simulink library "UserBlocks"  (R2014a)
settings: Solver=ode45  SolverMode=SingleTasking  StartTime=0.0  StopTime=10.0  RelTol=1e-3
values from neighbouring files (symbols this model uses):
  a = param.a    [DSC_Control_Analysis.m]    (also in DSC_Control_Analysis_Exp.m; DSC_Speed_Control_Analysis.m; EmpiricalTireCurves.m = 1.35; FFW_Fx.m = sqrt(curvature/(2*clothoidLength)))
  b = 1.15    [EmpiricalTireCurves.m]
  Cfls = Cfl    [EC_params_nissan.m]
  Crls = Crl    [EC_params_nissan.m]
  d0 = CSTR.d0    [Ext_MPCPara.m]
  freq = Fs/2*linspace(0,1,NFFT/2)    [AACplottingcode.m]    (also in If_alpha_tp_observer.m; If_alpha_tp_observer_for_c_code.m; If_alpha_tp_observer_shoreline.m)
  Iz = param.Iz    [DSC_Control_Analysis.m]    (also in DSC_Control_Analysis_Exp.m; DSC_Speed_Control_Analysis.m; EmpiricalTireCurves.m = 1300)
  K = 10    [EC_params_nissan.m]
  Ks = -10    [EC_params_nissan.m]
  Ksl = -10    [EC_params_nissan.m]
  Kt = 40000    [EC_params_nissan.m]
  Ku = -40000    [EC_params_nissan.m]
  m = 1724    [EmpiricalTireCurves.m]
  mu_s = mu_p    (= 0.6)    [EC_params_nissan.m]    (also in EmpiricalTireCurves.m = 0.55)
  Ns = 10    [EC_params_nissan.m]
  num = num+MTnum(m)    [Build_MtMuMy.m]
  q = 1    [EC_params_nissan.m]
  Taoh = CSTR.Taoh    [Ext_MPCPara.m]
  Ts = 0.002    [DSC_Control_Analysis.m]    (also in DSC_Control_Analysis_Exp.m; DSC_Speed_Control_Analysis.m; EC_params_nissan.m; Ext_MPCPara.m = SSD.Ts)
undefined symbols (not defined in the file or in its folder): acceAmp, ack, alphaFrontSteeringLimit, alphaFrontTable, bit, c, Cfl, Crl, CSTR, dden, deltaPsiDotGain, deltDist, den, denafilt, dnum, elaDotGain, filtera, filterb, frontAlphaLookup, frontForceLookup, FuelStartCalTime, FyFtable, gpsins, h, h_roll, hal_filter_den, hal_filter_num, hwx, hwy5, initAcce, initSpeed, isDriverNoise, lkparams, mapDataFull, mapMatchingParams, maxFrontForce, maxNumSegs, mdPtrs, numafilt, param, rearAlphaLookup, rfl, rfr, rrl, rrr, sglu, SIMP, simuCond, slimFxl, slimFxu, sliml, slimMll, slimMlr, slimMul, slimMur, slimu, sr, SSD, Standard, steering_limit ... (+7)
libraries: simulink x28, slrtlib x18, UserBlocks x6, slrtsoftinglib x6, MickLibBlocks x1, DriftControllerLibrary x1
(part 5 of 6)

== system UserBlocks/MPCACC/PIDACC/MPC MTCACC/MTC ACC control ==
  mdPtrs : Inport
  sysOuts : Inport  Port=2
  Prevel : Inport  Port=3
  VehVel : Inport  Port=4
  MPC CAN Receive1 : Subsystem  AncestorBlock=UserBlocks/MPC CAN Connection/MPC CAN Receive
  MPC CAN Send : Subsystem  AncestorBlock=UserBlocks/MPC CAN Connection/MPC CAN Send
  Samp2 : ZeroOrderHold  SampleTime=SSD.Ts
  Samp4 : ZeroOrderHold  SampleTime=SSD.Ts
  "Setup " : slrtsoftinglib/CAN-AC2-104 SJA 1000/Setup   board=1  can1Baudrate=500 kBaud  can1UserBR=[1,1,4,3]  can2Baudrate=500 kBaud  can2UserBR=[1,1,4,3]  init=[]  term=[]  bus_off_out=off  bus_off_rec=Off  ioBaseAddressL=0x240  memBaseAddressL=0xd0000  intNo=None
  T : Terminator
  Unit Delay : UnitDelay  SampleTime=SSD.Ts
  Ctrl : Outport
  epsilon : Outport  Port=2
  wires:
  MPC CAN Receive1/1(Ctrl) -> Ctrl/1, Unit Delay/1  "u(k)"
  MPC CAN Receive1/2(epsilon) -> epsilon/1
  Prevel/1 -> Samp4/1
  sysOuts/1 -> MPC CAN Send/2(sysOuts)
  VehVel/1 -> Samp2/1
  Unit Delay/1 -> MPC CAN Send/3(Ctrl)
  Samp4/1 -> MPC CAN Send/4(Prevel)
  Samp2/1 -> T/1
  mdPtrs/1 -> MPC CAN Send/1(mdPtrs)

== system UserBlocks/Steering Controller/HAL-9000/Double chirp/Chirp One ==
  note: freqSlope = deltaFreq/targetTime;
      | instantaneousFreq(t) = freqSlope*t + initialFreq;
      | intantaneousPhase(t) = integral(instFreq) = ...
      |       0.5*freqSlope*t^2 + initialFreq*t;
      | outputSignal(t) = sin(instantaneousPhase(t));
  Start Time : Inport
  Clock1 : Clock
      settings: DisableCoverage=on
  Gain : Gain  DisableCoverage=on  Gain=0.5  OutDataTypeStr=Inherit: Same as input  ParamDataTypeStr=Inherit: Same as input
  Output : Trigonometry
  Product : Product  DisableCoverage=on  Inputs=*/  SaturateOnIntegerOverflow=on  InputSameDT=on  OutDataTypeStr=Inherit: Same as first input
  Product1 : Product  DisableCoverage=on  SaturateOnIntegerOverflow=on  InputSameDT=on  OutDataTypeStr=Inherit: Same as first input
  Product2 : Product  DisableCoverage=on  SaturateOnIntegerOverflow=on  InputSameDT=on  OutDataTypeStr=Inherit: Same as first input
  Saturation : Saturate  UpperLimit=duration/2  LowerLimit=0
  Sum : Sum  DisableCoverage=on  Inputs=|++  SaturateOnIntegerOverflow=on  InputSameDT=on  OutDataTypeStr=Inherit: Same as first input
  Sum1 : Sum  DisableCoverage=on  Inputs=-+|  SaturateOnIntegerOverflow=on  InputSameDT=on  OutDataTypeStr=Inherit: Same as first input
  deltaFreq : Constant  DisableCoverage=on  Value=2*pi*(f2-f1)
  initialFreq : Constant  DisableCoverage=on  Value=2*pi*f1
  targetTime : Constant  DisableCoverage=on  Value=T
  Out2 : Outport
  wires:
  Saturation/1 -> Product2/1, Product1/1
  Output/1 -> Out2/1
  Product2/1 -> Output/1
  Sum/1 -> Product2/2
  initialFreq/1 -> Sum/2
  Product1/1 -> Sum/1
  Gain/1 -> Product1/2
  Product/1 -> Gain/1
  targetTime/1 -> Product/2
  deltaFreq/1 -> Product/1
  Start Time/1 -> Sum1/1
  Clock1/1 -> Sum1/2
  Sum1/1 -> Saturation/1

== system UserBlocks/Steering Controller/HAL-9000/Double chirp/Chirp Two ==
  note: freqSlope = deltaFreq/targetTime;
      | instantaneousFreq(t) = freqSlope*t + initialFreq;
      | intantaneousPhase(t) = integral(instFreq) = ...
      |       0.5*freqSlope*t^2 + initialFreq*t;
      | outputSignal(t) = sin(instantaneousPhase(t));
  Start Time : Inport
  Clock1 : Clock
      settings: DisableCoverage=on
  Gain : Gain  DisableCoverage=on  Gain=0.5  OutDataTypeStr=Inherit: Same as input  ParamDataTypeStr=Inherit: Same as input
  Output : Trigonometry
  Product : Product  DisableCoverage=on  Inputs=*/  SaturateOnIntegerOverflow=on  InputSameDT=on  OutDataTypeStr=Inherit: Same as first input
  Product1 : Product  DisableCoverage=on  SaturateOnIntegerOverflow=on  InputSameDT=on  OutDataTypeStr=Inherit: Same as first input
  Product2 : Product  DisableCoverage=on  SaturateOnIntegerOverflow=on  InputSameDT=on  OutDataTypeStr=Inherit: Same as first input
  Saturation : Saturate  UpperLimit=duration/2  LowerLimit=0
  Sum : Sum  DisableCoverage=on  Inputs=|++  SaturateOnIntegerOverflow=on  InputSameDT=on  OutDataTypeStr=Inherit: Same as first input
  Sum1 : Sum  DisableCoverage=on  Inputs=-+|  SaturateOnIntegerOverflow=on  InputSameDT=on  OutDataTypeStr=Inherit: Same as first input
  deltaFreq : Constant  DisableCoverage=on  Value=2*pi*(f2-f1)
  initialFreq : Constant  DisableCoverage=on  Value=2*pi*f1
  targetTime : Constant  DisableCoverage=on  Value=T
  Out2 : Outport
  wires:
  Saturation/1 -> Product2/1, Product1/1
  Output/1 -> Out2/1
  Product2/1 -> Output/1
  Sum/1 -> Product2/2
  initialFreq/1 -> Sum/2
  Product1/1 -> Sum/1
  Gain/1 -> Product1/2
  Product/1 -> Gain/1
  targetTime/1 -> Product/2
  deltaFreq/1 -> Product/1
  Start Time/1 -> Sum1/1
  Clock1/1 -> Sum1/2
  Sum1/1 -> Saturation/1

== system UserBlocks/TTS Steering Control/Compute Steering Along Path/StaticMap/Map-Matching Primatives Dynamic Map P1 ==
  States : Inport
  Map : Inport  Port=2
  3-second delay : Step  Time=3  SampleTime=0
  Bus Creator : BusCreator  Inputs=3
  Bus Selector : BusSelector  OutputSignals=Pos E,Pos N,Yaw Angle,Vx
  Constant : Constant  Value=0
  Constant1 : Constant  Value=pi/2  SampleTime=Ts
  Data Type Conversion : DataTypeConversion  OutDataTypeStr=double
  General Map-Matching Dynamic Map : Subsystem
  Logical Operator : Logic  Operator=OR  AllPortsSameDT=off  OutDataTypeStr=boolean
  Sum : Sum  Inputs=|++
  Unit Delay : UnitDelay  SampleTime=-1
  Match Out : Outport
  wires:
  Constant/1 -> General Map-Matching Dynamic Map/3(posU)
  Logical Operator/1 -> Data Type Conversion/1, Unit Delay/1
  Bus Selector/3 -> Sum/1  "<Yaw Angle>"
  Data Type Conversion/1 -> General Map-Matching Dynamic Map/6(enable)
  Unit Delay/1 -> Logical Operator/2
  3-second delay/1 -> Logical Operator/1
  Bus Selector/4 -> General Map-Matching Dynamic Map/5(vx_cg)  "<Vx>"
  General Map-Matching Dynamic Map/3(debugOut) -> Bus Creator/3  "debugOut"
  Sum/1 -> General Map-Matching Dynamic Map/4(yaw)
  Constant1/1 -> Sum/2
  General Map-Matching Dynamic Map/2(curOut) -> Bus Creator/2  "curOut"
  General Map-Matching Dynamic Map/1(matchOut) -> Bus Creator/1  "matchOut"
  States/1 -> Bus Selector/1
  Bus Selector/1 -> General Map-Matching Dynamic Map/1(posE)  "<Pos E>"
  Bus Selector/2 -> General Map-Matching Dynamic Map/2(posN)  "<Pos N>"
  Bus Creator/1 -> Match Out/1
  Map/1 -> General Map-Matching Dynamic Map/7(Map)

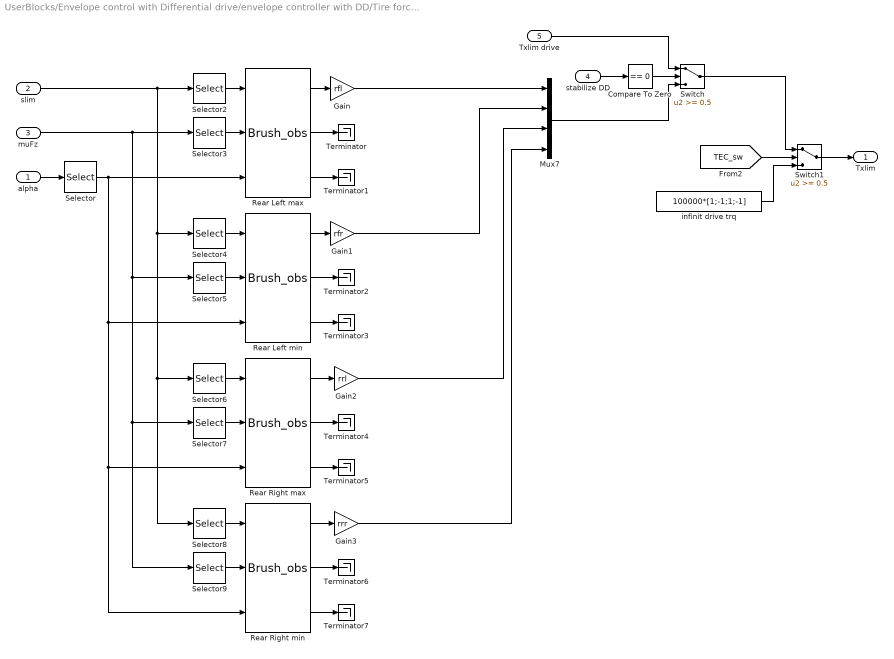
== system UserBlocks/Envelope control with Differential drive/envelope controller with DD/Tire force control/limit_cal/Fx_limit_cal ==
  alpha : Inport
  slim : Inport  Port=2
  muFz : Inport  Port=3
  stabilize DD : Inport  Port=4
  Txlim drive : Inport  Port=5
  Compare To Zero : simulink/Logic and Bit Operations/Compare To Zero  relop===  OutDataTypeStr=uint8  ZeroCross=off
  Gain : Gain  Gain=rfl
  Gain1 : Gain  Gain=rfr
  Gain2 : Gain  Gain=rrl
  Gain3 : Gain  Gain=rrr
  Mux7 : Mux
  Rear Left max : S-Function  FunctionName=Brush_obs  Parameters=Crl, Crls, l  EnableBusSupport=off
  Rear Left min : S-Function  FunctionName=Brush_obs  Parameters=Crl, Crls, l  EnableBusSupport=off
  Rear Right max : S-Function  FunctionName=Brush_obs  Parameters=Crr, Crrs, l  EnableBusSupport=off
  Rear Right min : S-Function  FunctionName=Brush_obs  Parameters=Crr, Crrs, l  EnableBusSupport=off
  Selector : Selector  InputPortWidth=2  Indices=2
  Selector2 : Selector  InputPortWidth=4
  Selector3 : Selector  InputPortWidth=4  Indices=3
  Selector4 : Selector  InputPortWidth=4  Indices=2
  Selector5 : Selector  InputPortWidth=4  Indices=3
  Selector6 : Selector  InputPortWidth=4  Indices=3
  Selector7 : Selector  InputPortWidth=4  Indices=4
  Selector8 : Selector  InputPortWidth=4  Indices=4
  Selector9 : Selector  InputPortWidth=4  Indices=4
  Switch : Switch  Threshold=0.5
  Switch1 : Switch  Threshold=0.5
  Terminator{,1..7} (8 alike) : Terminator
  infinit drive trq : Constant  Value=100000*[1;-1;1;-1]
  Txlim : Outport
  wires:
  Switch/1 -> Switch1/1
  Txlim drive/1 -> Switch/1
  Mux7/1 -> Switch/3
  stabilize DD/1 -> Compare To Zero/1
  Compare To Zero/1 -> Switch/2
  infinit drive trq/1 -> Switch1/3
  Switch1/1 -> Txlim/1
  [TEC_sw] -> Switch1/2
  Gain2/1 -> Mux7/3
  Gain/1 -> Mux7/1
  alpha/1 -> Selector/1
  Selector2/1 -> Rear Left max/1
  Selector3/1 -> Rear Left max/2
  Selector4/1 -> Rear Left min/1
  Selector5/1 -> Rear Left min/2
  Selector6/1 -> Rear Right max/1
  Selector7/1 -> Rear Right max/2
  Selector8/1 -> Rear Right min/1
  Selector9/1 -> Rear Right min/2
  slim/1 -> Selector2/1, Selector4/1, Selector8/1, Selector6/1
  muFz/1 -> Selector3/1, Selector5/1, Selector9/1, Selector7/1
  Selector/1 -> Rear Left max/3, Rear Left min/3, Rear Right min/3, Rear Right max/3
  Rear Left max/2 -> Terminator/1
  Rear Left max/3 -> Terminator1/1
  Rear Left min/2 -> Terminator2/1
  Rear Left min/3 -> Terminator3/1
  Rear Right max/2 -> Terminator4/1
  Rear Right max/3 -> Terminator5/1
  Rear Right min/2 -> Terminator6/1
  Rear Right min/3 -> Terminator7/1
  Rear Left max/1 -> Gain/1
  Rear Left min/1 -> Gain1/1
  Rear Right max/1 -> Gain2/1
  Rear Right min/1 -> Gain3/1
  Gain1/1 -> Mux7/2
  Gain3/1 -> Mux7/4

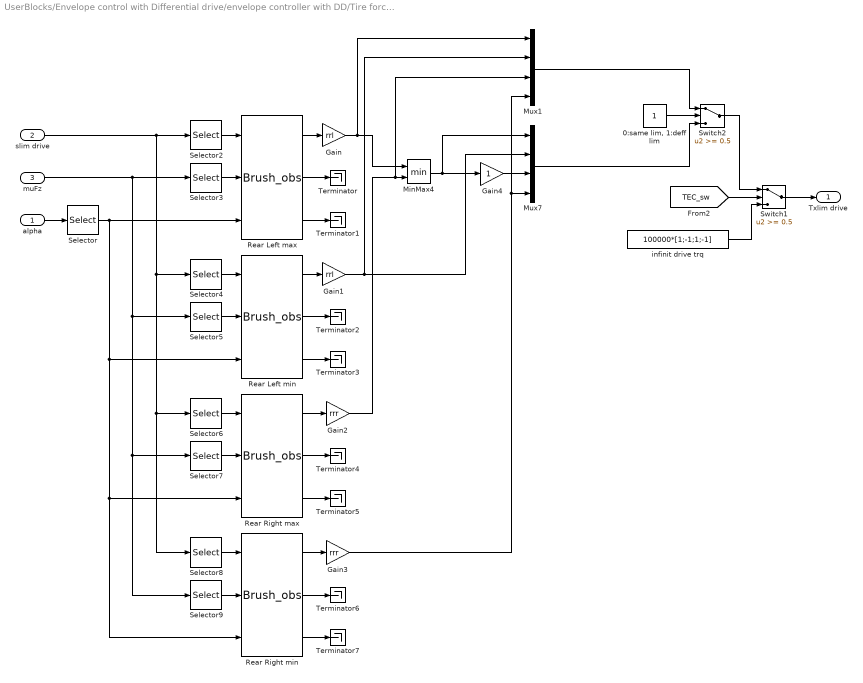
== system UserBlocks/Envelope control with Differential drive/envelope controller with DD/Tire force control/limit_cal/Fx_limit_cal1 ==
  alpha : Inport
  slim drive : Inport  Port=2
  muFz : Inport  Port=3
  "0:same lim, 1:deff lim" : Constant
  Gain : Gain  Gain=rrl
  Gain1 : Gain  Gain=rrl
  Gain2 : Gain  Gain=rrr
  Gain3 : Gain  Gain=rrr
  Gain4 : Gain
  MinMax4 : MinMax  Inputs=2
  Mux1 : Mux
  Mux7 : Mux
  Rear Left max : S-Function  FunctionName=Brush_obs  Parameters=Crl, Crls, l  EnableBusSupport=off
  Rear Left min : S-Function  FunctionName=Brush_obs  Parameters=Crl, Crls, l  EnableBusSupport=off
  Rear Right max : S-Function  FunctionName=Brush_obs  Parameters=Crr, Crrs, l  EnableBusSupport=off
  Rear Right min : S-Function  FunctionName=Brush_obs  Parameters=Crr, Crrs, l  EnableBusSupport=off
  Selector : Selector  InputPortWidth=2  Indices=2
  Selector2 : Selector  InputPortWidth=4
  Selector3 : Selector  InputPortWidth=4  Indices=3
  Selector4 : Selector  InputPortWidth=4  Indices=2
  Selector5 : Selector  InputPortWidth=4  Indices=3
  Selector6 : Selector  InputPortWidth=4  Indices=3
  Selector7 : Selector  InputPortWidth=4  Indices=4
  Selector8 : Selector  InputPortWidth=4  Indices=4
  Selector9 : Selector  InputPortWidth=4  Indices=4
  Switch1 : Switch  Threshold=0.5
  Switch2 : Switch  Threshold=0.5
  Terminator{,1..7} (8 alike) : Terminator
  infinit drive trq : Constant  Value=100000*[1;-1;1;-1]
  Txlim drive : Outport
  wires:
  "0:same lim, 1:deff lim"/1 -> Switch2/2
  Switch2/1 -> Switch1/1
  Mux1/1 -> Switch2/1
  Mux7/1 -> Switch2/3
  Gain4/1 -> Mux7/3
  Gain/1 -> Mux1/1, MinMax4/1
  MinMax4/1 -> Gain4/1, Mux7/1
  Switch1/1 -> Txlim drive/1
  infinit drive trq/1 -> Switch1/3
  [TEC_sw] -> Switch1/2
  Gain3/1 -> Mux1/4, Mux7/4
  Gain1/1 -> Mux1/2, Mux7/2
  Rear Right min/1 -> Gain3/1
  Rear Right max/1 -> Gain2/1
  Rear Left min/1 -> Gain1/1
  Rear Left max/1 -> Gain/1
  Rear Right min/3 -> Terminator7/1
  Rear Right min/2 -> Terminator6/1
  Rear Right max/3 -> Terminator5/1
  Rear Right max/2 -> Terminator4/1
  Rear Left min/3 -> Terminator3/1
  Rear Left min/2 -> Terminator2/1
  Rear Left max/3 -> Terminator1/1
  Rear Left max/2 -> Terminator/1
  Selector/1 -> Rear Right max/3, Rear Right min/3, Rear Left min/3, Rear Left max/3
  muFz/1 -> Selector7/1, Selector9/1, Selector5/1, Selector3/1
  slim drive/1 -> Selector6/1, Selector8/1, Selector4/1, Selector2/1
  Selector9/1 -> Rear Right min/2
  Selector8/1 -> Rear Right min/1
  Selector7/1 -> Rear Right max/2
  Selector6/1 -> Rear Right max/1
  Selector5/1 -> Rear Left min/2
  Selector4/1 -> Rear Left min/1
  Selector3/1 -> Rear Left max/2
  Selector2/1 -> Rear Left max/1
  alpha/1 -> Selector/1
  Gain2/1 -> Mux1/3, MinMax4/2

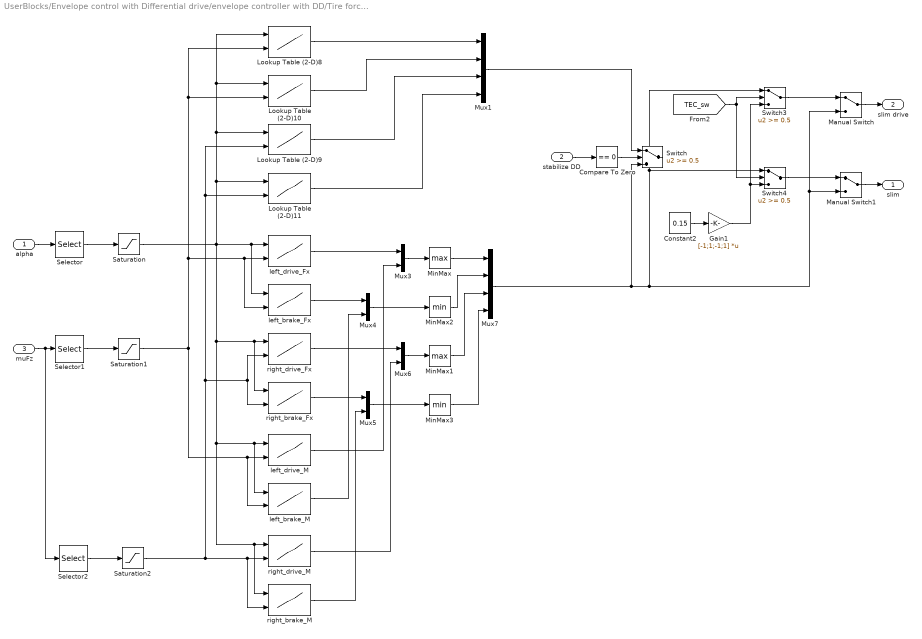
== system UserBlocks/Envelope control with Differential drive/envelope controller with DD/Tire force control/limit_cal/slip_limit_cal1 ==
  alpha : Inport
  stabilize DD : Inport  Port=2
  muFz : Inport  Port=3
  Compare To Zero : simulink/Logic and Bit Operations/Compare To Zero  relop===  OutDataTypeStr=uint8  ZeroCross=off
  Constant2 : Constant  Value=0.15
  Gain1 : Gain  Gain=[-1;1;-1;1]  Multiplication=Matrix(K*u)
  Lookup Table (2-D)10 : Lookup2D  RowIndex=limitcal_alphatbl  ColumnIndex=limitcal_muFztbl  Table=slimu  SampleTime=0.002
  Lookup Table (2-D)11 : Lookup2D  RowIndex=limitcal_alphatbl  ColumnIndex=limitcal_muFztbl  Table=slimu  SampleTime=0.002
  Lookup Table (2-D)8 : Lookup2D  RowIndex=limitcal_alphatbl  ColumnIndex=limitcal_muFztbl  Table=sliml  SampleTime=0.002
  Lookup Table (2-D)9 : Lookup2D  RowIndex=limitcal_alphatbl  ColumnIndex=limitcal_muFztbl  Table=sliml  SampleTime=0.002
  Manual Switch : ManualSwitch
  Manual Switch1 : ManualSwitch
  MinMax : MinMax  Function=max
  MinMax1 : MinMax  Function=max
  MinMax2 : MinMax
  MinMax3 : MinMax
  Mux1 : Mux
  Mux{3..6} (4 alike) : Mux  Inputs=2
  Mux7 : Mux
  Saturation : Saturate  UpperLimit=40/180*pi  LowerLimit=-40/180*pi
  Saturation1 : Saturate  UpperLimit=6000  LowerLimit=1
  Saturation2 : Saturate  UpperLimit=6000  LowerLimit=1
  Selector : Selector  InputPortWidth=2  Indices=2
  Selector1 : Selector  InputPortWidth=4  Indices=3
  Selector2 : Selector  InputPortWidth=4  Indices=4
  Switch : Switch  Threshold=0.5
  Switch3 : Switch  Threshold=0.5
  Switch4 : Switch  Threshold=0.5
  left_brake_Fx : Lookup2D  RowIndex=limitcal_alphatbl  ColumnIndex=limitcal_muFztbl  Table=slimFxu  SampleTime=0.002
  left_brake_M : Lookup2D  RowIndex=limitcal_alphatbl  ColumnIndex=limitcal_muFztbl  Table=slimMul  SampleTime=0.002
  left_drive_Fx : Lookup2D  RowIndex=limitcal_alphatbl  ColumnIndex=limitcal_muFztbl  Table=slimFxl  SampleTime=0.002
  left_drive_M : Lookup2D  RowIndex=limitcal_alphatbl  ColumnIndex=limitcal_muFztbl  Table=slimMll  SampleTime=0.002
  right_brake_Fx : Lookup2D  RowIndex=limitcal_alphatbl  ColumnIndex=limitcal_muFztbl  Table=slimFxu  SampleTime=0.002
  right_brake_M : Lookup2D  RowIndex=limitcal_alphatbl  ColumnIndex=limitcal_muFztbl  Table=slimMur  SampleTime=0.002
  right_drive_Fx : Lookup2D  RowIndex=limitcal_alphatbl  ColumnIndex=limitcal_muFztbl  Table=slimFxl  SampleTime=0.002
  right_drive_M : Lookup2D  RowIndex=limitcal_alphatbl  ColumnIndex=limitcal_muFztbl  Table=slimMlr  SampleTime=0.002
  slim : Outport
  slim drive : Outport  Port=2
  wires:
  Mux1/1 -> Switch/1
  Switch4/1 -> Manual Switch1/1
  Switch3/1 -> Manual Switch/1
  Manual Switch/1 -> slim drive/1
  Manual Switch1/1 -> slim/1
  Gain1/1 -> Switch4/3, Switch3/3
  [TEC_sw] -> Switch4/2, Switch3/2
  stabilize DD/1 -> Compare To Zero/1
  Constant2/1 -> Gain1/1
  Saturation2/1 -> right_brake_M/2, right_drive_M/2, right_brake_Fx/2, right_drive_Fx/2, Lookup Table (2-D)9/2, Lookup Table (2-D)11/2
  Saturation1/1 -> left_brake_M/2, left_drive_M/2, left_brake_Fx/2, left_drive_Fx/2, Lookup Table (2-D)8/2, Lookup Table (2-D)10/2
  Saturation/1 -> left_brake_Fx/1, left_drive_Fx/1, right_brake_Fx/1, right_drive_Fx/1, right_brake_M/1, right_drive_M/1, left_brake_M/1, left_drive_M/1, Lookup Table (2-D)8/1, Lookup Table (2-D)10/1, Lookup Table (2-D)9/1, Lookup Table (2-D)11/1
  right_brake_Fx/1 -> Mux5/1
  right_brake_M/1 -> Mux5/2
  right_drive_M/1 -> Mux6/2
  Selector2/1 -> Saturation2/1
  MinMax3/1 -> Mux7/4
  MinMax1/1 -> Mux7/3
  MinMax2/1 -> Mux7/2
  MinMax/1 -> Mux7/1
  Mux5/1 -> MinMax3/1
  Mux4/1 -> MinMax2/1
  Mux6/1 -> MinMax1/1
  Mux3/1 -> MinMax/1
  left_brake_M/1 -> Mux4/2
  left_drive_M/1 -> Mux3/2
  right_drive_Fx/1 -> Mux6/1
  left_brake_Fx/1 -> Mux4/1
  left_drive_Fx/1 -> Mux3/1
  Selector/1 -> Saturation/1
  Selector1/1 -> Saturation1/1
  muFz/1 -> Selector2/1, Selector1/1
  alpha/1 -> Selector/1
  Compare To Zero/1 -> Switch/2
  Lookup Table (2-D)8/1 -> Mux1/1
  Lookup Table (2-D)10/1 -> Mux1/2
  Lookup Table (2-D)9/1 -> Mux1/3
  Lookup Table (2-D)11/1 -> Mux1/4
  Mux7/1 -> Switch4/1, Switch3/1, Manual Switch/2, Manual Switch1/2, Switch/3

== system UserBlocks/Envelope control with Differential drive/envelope controller with DD/Tire force control/s_cal /prevent zero ==
  In1 : Inport
  Abs : Abs
  Constant : Constant  Value=1/3.6
  Product : Product  RndMeth=Zero
  Relational Operator : RelationalOperator  Operator=>  OutDataTypeStr=boolean
  Sign : Signum
  Switch : Switch  Threshold=0.5
  Switch1 : Switch  Threshold=0.5
  Unit Delay : UnitDelay  InitialCondition=1  SampleTime=Ts
  Out1 : Outport
  wires:
  Switch/1 -> Out1/1
  Relational Operator/1 -> Switch/2, Switch1/2
  Constant/1 -> Relational Operator/2, Product/1
  Abs/1 -> Relational Operator/1
  In1/1 -> Switch/1, Abs/1, Sign/1
  Sign/1 -> Switch1/1
  Product/1 -> Switch/3
  Switch1/1 -> Product/2, Unit Delay/1
  Unit Delay/1 -> Switch1/3

== system UserBlocks/Envelope control with Differential drive/envelope controller with DD/Tire force control/s_cal /prevent zero1 ==
  In1 : Inport
  Abs : Abs
  Constant : Constant  Value=1/3.6
  Product : Product  RndMeth=Zero
  Relational Operator : RelationalOperator  Operator=>  OutDataTypeStr=boolean
  Sign : Signum
  Switch : Switch  Threshold=0.5
  Switch1 : Switch  Threshold=0.5
  Unit Delay : UnitDelay  InitialCondition=1  SampleTime=Ts
  Out1 : Outport
  wires:
  Unit Delay/1 -> Switch1/3
  Switch1/1 -> Unit Delay/1, Product/2
  Product/1 -> Switch/3
  Sign/1 -> Switch1/1
  In1/1 -> Sign/1, Abs/1, Switch/1
  Abs/1 -> Relational Operator/1
  Constant/1 -> Product/1, Relational Operator/2
  Relational Operator/1 -> Switch1/2, Switch/2
  Switch/1 -> Out1/1

== system UserBlocks/Envelope control with Differential drive/envelope controller with DD/Tire force control/steering control/delta limit cal ==
  Vx : Inport
  beta : Inport  Port=2
  yaw rate : Inport  Port=3
  aflim : Inport  Port=4
  Fcn : Fcn  Expr=u[1]+a/u[3]*u[2]+u[4]  SampleTime=0.002
  Fcn1 : Fcn  Expr=u[1]+a/u[3]*u[2]-u[4]  SampleTime=0.002
  Mux : Mux
  upper lim : Outport
  lower lim : Outport  Port=2
  wires:
  beta/1 -> Mux/1
  yaw rate/1 -> Mux/2
  aflim/1 -> Mux/4
  Vx/1 -> Mux/3
  Fcn1/1 -> lower lim/1
  Fcn/1 -> upper lim/1
  Mux/1 -> Fcn/1, Fcn1/1

== system UserBlocks/Envelope control with Differential drive/envelope controller with DD/vehicle motion control/EC/ay_limit_cal ==
  peak_force_hat : Inport
  drive_trq : Inport  Port=2
  ExpSW : Inport  Port=3
  Constant : Constant  Value=0
  Constant1 : Constant  Value=1.75
  Demux : Demux
  Demux1 : Demux  Outputs=2
  Fcn : Fcn  Expr=u(1)*u(1)-u(2)*u(2)
  Fcn1 : Fcn  Expr=u(1)*u(1)-u(2)*u(2)
  Gain : Gain  Gain=1100
  Gain1 : Gain  Gain=400
  Gain2 : Gain  Gain=a
  Gain3 : Gain  Gain=b
  Gain4 : Gain  Gain=1+b/a
  Gain5 : Gain  Gain=1+a/b
  Gain6 : Gain  Gain=1/m
  Gain7 : Gain  Gain=1/rrl
  Gain8 : Gain  Gain=1/rrr
  Math Function : Math  Operator=sqrt  SaturateOnIntegerOverflow=on
  Math Function1 : Math  Operator=sqrt  SaturateOnIntegerOverflow=on
  MinMax : MinMax  Function=max  Inputs=2
  MinMax1 : MinMax  Function=max  Inputs=2
  Mux : Mux  Inputs=2
  Mux1 : Mux  Inputs=2
  Mux4 : Mux  Inputs=2
  Sum : Sum  Inputs=|++
  Sum1 : Sum  Inputs=|+-
  Sum2 : Sum  Inputs=|++
  Sum3 : Sum  Inputs=-|+
  Switch : Switch
  Switch1 : Switch
  Switch2 : Switch  Threshold=0.5
  Driving force : Outport
  ay_limit : Outport  Port=2
  wires:
  Mux4/1 -> Driving force/1
  Gain8/1 -> Mux4/2, Mux1/2
  Gain7/1 -> Mux4/1, Mux/2
  ExpSW/1 -> Switch2/2
  Switch/1 -> Switch2/1
  Switch2/1 -> Demux1/1
  Gain6/1 -> ay_limit/1
  Switch1/1 -> Gain6/1
  Gain4/1 -> Switch1/3
  Gain5/1 -> Switch1/1
  Gain3/1 -> Sum3/2
  Gain2/1 -> Sum3/1
  Sum3/1 -> Switch1/2
  Sum2/1 -> Gain4/1, Gain3/1
  Sum/1 -> Gain5/1, Gain2/1
  Math Function1/1 -> Sum2/2
  Math Function/1 -> Sum2/1
  Gain1/1 -> Switch/3
  Gain/1 -> Switch/1
  Sum1/1 -> Gain1/1, Gain/1, Switch/2
  Constant1/1 -> Sum1/2
  drive_trq/1 -> Switch2/3, Sum1/1
  MinMax1/1 -> Math Function1/1
  MinMax/1 -> Math Function/1
  Constant/1 -> MinMax/2, MinMax1/2
  Fcn/1 -> MinMax/1
  Fcn1/1 -> MinMax1/1
  Mux1/1 -> Fcn1/1
  Demux1/2 -> Gain8/1
  Demux1/1 -> Gain7/1
  Demux/4 -> Mux1/1
  Demux/3 -> Mux/1
  Mux/1 -> Fcn/1
  Demux/2 -> Sum/2
  Demux/1 -> Sum/1
  peak_force_hat/1 -> Demux/1

== system UserBlocks/LQACC/PIDACC/Car-Following System/Car-Follow Sys/Des Dist ==
  Vf : Inport
  D0 : Constant  Value=d0
  Sum1 : Sum  SaturateOnIntegerOverflow=on
  Th : Gain  Gain=Taoh  SaturateOnIntegerOverflow=on  OutDataTypeStr=Inherit: Same as input  ParamDataTypeStr=Inherit: Same as input
  DesDist : Outport
  wires:
  Vf/1 -> Th/1
  Th/1 -> Sum1/1
  D0/1 -> Sum1/2
  Sum1/1 -> DesDist/1

== system UserBlocks/LQACC/PIDACC/MPC MTCACC/MTC ACC control/LQ controller1 ==
  PreAcce : Inport
  sysOuts : Inport  Port=2
  Kx : Gain  Gain="[0.2236    0.5767   -0.7384]"  Multiplication=Matrix(K*u) (u vector)
  Sat : Saturate  UpperLimit=CSTR.uMax  LowerLimit=CSTR.uMin
  Terminator : Terminator
  e : Constant  Value=0
  desAccel : Outport
  epsilon : Outport  Port=2
  wires:
  e/1 -> epsilon/1
  Kx/1 -> Sat/1  "u(k)"
  PreAcce/1 -> Terminator/1
  sysOuts/1 -> Kx/1
  Sat/1 -> desAccel/1

== system UserBlocks/LQACC/PIDACC/PreVehicle/City Road StartTime=20s/DirverNoise ==
  In : Inport
  Band-Limited White Noise : simulink/Sources/Band-Limited White Noise  Cov=[0.0001*isDriverNoise]  Ts=0.1  seed=[23341]
  Mux1 : Mux  Inputs=2
  Scope : Scope
      settings: SaveName=ScopeData7
  Sum : Sum  Inputs=|++
  TFcn1 : TransferFcn  Denominator=[0.7 1]
  Out : Outport
  wires:
  TFcn1/1 -> Sum/2
  Mux1/1 -> Scope/1
  Sum/1 -> Mux1/1, Out/1
  In/1 -> Mux1/2, Sum/1
  Band-Limited White Noise/1 -> TFcn1/1

== system UserBlocks/LQACC/PIDACC/PreVehicle/City Road StartTime=20s/Modification ==
  in : Inport
  Delay : TransportDelay  DelayTime=10  InitialOutput=5
  MinMax : MinMax  Function=max  Inputs=2
  Step : Step  Time=20  Before=5  After=0  SampleTime=0
  Out : Outport
  wires:
  Delay/1 -> MinMax/1
  MinMax/1 -> Out/1
  in/1 -> Delay/1
  Step/1 -> MinMax/2

== system UserBlocks/LQACC/PIDACC/PreVehicle/City Road StartTime=20s/initSlope1 ==
  Xin : Inport
  ACCScope2 : Scope  NumInputPorts=2
      settings: YMin=-2~0  YMax=2~40  SaveName=ScopeData6
  ConstVp : Constant  Value=5
  Mux6 : Mux  Inputs=2
  ROperator : RelationalOperator  Operator=<=  OutDataTypeStr=boolean
  Ramp1 : simulink/Sources/Ramp  slope=initAcce  start=0  X0=initSpeed
  Switch3 : Switch  Threshold=0.5
  Xout : Outport
  wires:
  Mux6/1 -> ACCScope2/1
  ConstVp/1 -> ROperator/1
  Ramp1/1 -> Mux6/2, Switch3/3, ROperator/2
  ROperator/1 -> Switch3/2
  Xin/1 -> Mux6/1, Switch3/1
  Switch3/1 -> ACCScope2/2, Xout/1

== system UserBlocks/LQACC/PIDACC/PreVehicle/Express Way StartTime=20s/DirverNoise ==
  In : Inport
  Band-Limited White Noise : simulink/Sources/Band-Limited White Noise  Cov=[0.0001*isDriverNoise]  Ts=0.1  seed=[23341]
  Mux1 : Mux  Inputs=2
  Scope : Scope
      settings: SaveName=ScopeData7
  Sum : Sum  Inputs=|++
  TFcn1 : TransferFcn  Denominator=[0.7 1]
  Out : Outport
  wires:
  TFcn1/1 -> Sum/2
  Mux1/1 -> Scope/1
  Sum/1 -> Mux1/1, Out/1
  In/1 -> Mux1/2, Sum/1
  Band-Limited White Noise/1 -> TFcn1/1

== system UserBlocks/LQACC/PIDACC/PreVehicle/Express Way StartTime=20s/Modification ==
  in : Inport
  Delay : TransportDelay  DelayTime=10  InitialOutput=5
  MinMax : MinMax  Function=max  Inputs=2
  Step : Step  Time=25  Before=5  After=0  SampleTime=0
  Out : Outport
  wires:
  Delay/1 -> MinMax/1
  MinMax/1 -> Out/1
  in/1 -> Delay/1
  Step/1 -> MinMax/2

== system UserBlocks/LQACC/PIDACC/PreVehicle/Express Way StartTime=20s/initSlope1 ==
  Xin : Inport
  ACCScope2 : Scope  NumInputPorts=2
      settings: YMin=-2~0  YMax=2~40  SaveName=ScopeData6
  ConstVp : Constant  Value=5
  Mux6 : Mux  Inputs=2
  ROperator : RelationalOperator  Operator=<=  OutDataTypeStr=boolean
  Ramp1 : simulink/Sources/Ramp  slope=initAcce  start=0  X0=initSpeed
  Switch3 : Switch  Threshold=0.5
  Xout : Outport
  wires:
  Mux6/1 -> ACCScope2/1
  ConstVp/1 -> ROperator/1
  Ramp1/1 -> Mux6/2, Switch3/3, ROperator/2
  ROperator/1 -> Switch3/2
  Xin/1 -> Mux6/1, Switch3/1
  Switch3/1 -> ACCScope2/2, Xout/1

== system UserBlocks/MPCACC/PIDACC/Car-Following System/Car-Follow Sys/Des Dist ==
  Vf : Inport
  D0 : Constant  Value=d0
  Sum1 : Sum  SaturateOnIntegerOverflow=on
  Th : Gain  Gain=Taoh  SaturateOnIntegerOverflow=on  OutDataTypeStr=Inherit: Same as input  ParamDataTypeStr=Inherit: Same as input
  DesDist : Outport
  wires:
  Sum1/1 -> DesDist/1
  D0/1 -> Sum1/2
  Th/1 -> Sum1/1
  Vf/1 -> Th/1

== system UserBlocks/MPCACC/PIDACC/MPC MTCACC/MTC ACC control/MPC CAN Receive1 ==
  "CAN bit-unpacking " : slrtlib/CAN/Utilities/CAN bit-unpacking   bitpatterns={ [0:15],[16:31] }  dtypes={ 'int16' ,'int16'}
  Convert : DataTypeConversion  OutDataTypeStr=double
  Convert1 : DataTypeConversion  OutDataTypeStr=double
  Gain : Gain  Gain=.001
  "Receive " : slrtsoftinglib/CAN-AC2-104 SJA 1000/Receive   board=1  canPort=CAN 1  range=Standard (11-bit)  ids=[501]  lengths=[8]  output=Data  inten=off  ts=0.002  ididx=[0]
  Ctrl : Outport
  epsilon : Outport  Port=2
  wires:
  "CAN bit-unpacking "/2 -> Convert1/1
  "CAN bit-unpacking "/1 -> Convert/1
  "Receive "/1 -> "CAN bit-unpacking "/1
  Convert1/1 -> epsilon/1
  Convert/1 -> Gain/1
  Gain/1 -> Ctrl/1

== system UserBlocks/MPCACC/PIDACC/MPC MTCACC/MTC ACC control/MPC CAN Send ==
  mdPtrs : Inport
  sysOuts : Inport  Port=2
  Ctrl : Inport  Port=3
  Prevel : Inport  Port=4
  Bus Selector : BusSelector  OutputSignals=signal1,signal2,axCG
  Samp1 : ZeroOrderHold  SampleTime=SSD.Ts
  Samp2 : ZeroOrderHold  SampleTime=SSD.Ts
  Samp5 : ZeroOrderHold  SampleTime=SSD.Ts
  Subsystem : Subsystem
  wires:
  Samp2/1 -> Subsystem/4(In4)
  Samp1/1 -> Subsystem/3(In3)
  Samp5/1 -> Subsystem/2(In2)
  mdPtrs/1 -> Subsystem/1(In1)
  sysOuts/1 -> Bus Selector/1
  Bus Selector/1 -> Samp5/1  "<signal1>"
  Bus Selector/2 -> Samp1/1  "<signal2>"
  Bus Selector/3 -> Samp2/1  "<axCG>"
  Ctrl/1 -> Subsystem/5(In5)
  Prevel/1 -> Subsystem/6(In6)

== system UserBlocks/TTS Steering Control/Compute Steering Along Path/StaticMap/Map-Matching Primatives Dynamic Map P1/General Map-Matching Dynamic Map ==
  posE : Inport
  posN : Inport  Port=2
  posU : Inport  Port=3
  yaw : Inport  Port=4
  vx_cg : Inport  Port=5
  enable : Inport  Port=6
  Map : Inport  Port=7
  Bus Creator4 : BusCreator  Inputs=5
  Bus Creator5 : BusCreator  Inputs=6
  Bus Creator6 : BusCreator  Inputs=11
  Bus Selector : BusSelector  OutputSignals=segNum,segLength,kStart,kEnd,maxV,frictionBase,grade,bank,segType,segModType
  Demux2 : Demux  Outputs=5
  Demux4 : Demux  Outputs=11
  Demux6 : Demux  Outputs=6
  Get Segment Info Dynamic Map : Subsystem
  Mux : Mux  Inputs=11
  Mux1 : Mux  Inputs=5
  Terminator1 : Terminator
  Terminator2 : Terminator
  mapMatchingPrimitives Dynamic Map : Subsystem
  matchOut : Outport
  curOut : Outport  Port=2
  debugOut : Outport  Port=3
  wires:
  mapMatchingPrimitives Dynamic Map/2(e) -> Mux1/1  "e"
  mapMatchingPrimitives Dynamic Map/3(deltaPsi) -> Mux1/2  "dPsi"
  mapMatchingPrimitives Dynamic Map/4(curvature) -> Mux1/3  "crv"
  mapMatchingPrimitives Dynamic Map/7(isFinalSegment) -> Mux1/4  "finalSeg"
  mapMatchingPrimitives Dynamic Map/5(distanceToEnd) -> Mux1/5  "dst2end"
  mapMatchingPrimitives Dynamic Map/8(debugOut) -> Demux6/1  "debugOut"
  posE/1 -> mapMatchingPrimitives Dynamic Map/1(posE)
  posN/1 -> mapMatchingPrimitives Dynamic Map/2(posN)
  yaw/1 -> mapMatchingPrimitives Dynamic Map/3(yawAngle)
  posU/1 -> Terminator1/1
  vx_cg/1 -> Terminator2/1
  enable/1 -> mapMatchingPrimitives Dynamic Map/4(enable)
  Demux2/2 -> Bus Creator4/2  "dPsi"
  Mux/1 -> Demux4/1  "curOut"
  Bus Creator5/1 -> debugOut/1
  Bus Creator6/1 -> curOut/1
  Bus Creator4/1 -> matchOut/1
  Demux4/9 -> Bus Creator6/9  "curBank"
  Demux4/8 -> Bus Creator6/8  "curGrade"
  Demux4/7 -> Bus Creator6/7  "curFricCoef"
  Demux4/6 -> Bus Creator6/6  "curMaxV"
  Demux4/5 -> Bus Creator6/5  "curSegProg"
  Demux4/4 -> Bus Creator6/4  "curCrvF"
  Demux4/3 -> Bus Creator6/3  "curCrvI"
  Demux4/2 -> Bus Creator6/2  "curSegLngth"
  Demux4/1 -> Bus Creator6/1  "curSegNum"
  Demux2/5 -> Bus Creator4/5  "dst2end"
  Demux2/4 -> Bus Creator4/4  "finalSeg"
  Demux2/3 -> Bus Creator4/3  "crv"
  Demux2/1 -> Bus Creator4/1  "e"
  Demux6/6 -> Bus Creator5/6  "zErr"
  Demux6/5 -> Bus Creator5/5  "guessDist"
  Demux6/4 -> Bus Creator5/4  "enable"
  Demux6/3 -> Bus Creator5/3  "resErr"
  Demux6/2 -> Bus Creator5/2  "wasMax"
  Demux6/1 -> Bus Creator5/1  "numIter"
  Mux1/1 -> Demux2/1  "matchOut"
  Bus Selector/1 -> Mux/1  "<segNum>"
  Bus Selector/2 -> Mux/2  "<segLength>"
  Bus Selector/3 -> Mux/3  "<kStart>"
  Bus Selector/4 -> Mux/4  "<kEnd>"
  mapMatchingPrimitives Dynamic Map/1(seg) -> Get Segment Info Dynamic Map/1(segmentNumber)
  Get Segment Info Dynamic Map/1(segInfo) -> Bus Selector/1
  Bus Selector/5 -> Mux/6  "<maxV>"
  Bus Selector/6 -> Mux/7  "<frictionBase>"
  Bus Selector/7 -> Mux/8  "<grade>"
  Bus Selector/8 -> Mux/9  "<bank>"
  mapMatchingPrimitives Dynamic Map/6(currentSegmentProgress) -> Mux/5
  Bus Selector/9 -> Mux/10  "<segType>"
  Demux4/10 -> Bus Creator6/10  "curSegType"
  Map/1 -> Get Segment Info Dynamic Map/2(Map), mapMatchingPrimitives Dynamic Map/5(Map)
  Bus Selector/10 -> Mux/11  "<segModType>"
  Demux4/11 -> Bus Creator6/11  "curSegModType"

== system UserBlocks/MPCACC/PIDACC/MPC MTCACC/MTC ACC control/MPC CAN Send/Subsystem ==
  In1 : Inport
  In2 : Inport  Port=2
  In3 : Inport  Port=3
  In4 : Inport  Port=4
  In5 : Inport  Port=5
  In6 : Inport  Port=6
  "CAN bit-packing " : slrtlib/CAN/Utilities/CAN bit-packing   bitpatterns={ [0:7],[8:15],[16:23],[24,39],[40:55],[56:63] }
  Data Type Conversion1 : DataTypeConversion  OutDataTypeStr=int16  RndMeth=Nearest  SaturateOnIntegerOverflow=on
  Data Type Conversion{2..3,6..7} (4 alike) : DataTypeConversion  OutDataTypeStr=uint8  RndMeth=Nearest  SaturateOnIntegerOverflow=on
  Data Type Conversion4 : DataTypeConversion  OutDataTypeStr=int16  RndMeth=Nearest  SaturateOnIntegerOverflow=on
  Gain1 : Gain  Gain=1000
  Gain2 : Gain  Gain=10
  Gain3 : Gain  Gain=1000
  Gain4 : Gain  Gain=10
  Rate Transition1 : RateTransition
  Rate Transition3-relVel : RateTransition
  Rate Transition4-vehACCE : RateTransition
  Rate Transition5-distErr : RateTransition
  "Send " : slrtsoftinglib/CAN-AC2-104 SJA 1000/Send   board=1  canPort=CAN 1  range=Standard (11-bit)  ids=[500]  sizes=[8]  output=off  ts=0.01  ididx=[0]
  wires:
  In6/1 -> Gain4/1
  In5/1 -> Gain3/1
  In4/1 -> Rate Transition4-vehACCE/1
  In3/1 -> Rate Transition3-relVel/1
  In2/1 -> Rate Transition5-distErr/1
  In1/1 -> Rate Transition1/1
  Data Type Conversion2/1 -> "CAN bit-packing "/1
  "CAN bit-packing "/1 -> "Send "/1
  Rate Transition1/1 -> Data Type Conversion2/1
  Rate Transition5-distErr/1 -> Data Type Conversion3/1
  Rate Transition3-relVel/1 -> Gain2/1
  Rate Transition4-vehACCE/1 -> Gain1/1
  Data Type Conversion3/1 -> "CAN bit-packing "/2
  Data Type Conversion6/1 -> "CAN bit-packing "/3
  Data Type Conversion1/1 -> "CAN bit-packing "/4
  Data Type Conversion4/1 -> "CAN bit-packing "/5
  Data Type Conversion7/1 -> "CAN bit-packing "/6
  Gain3/1 -> Data Type Conversion4/1
  Gain1/1 -> Data Type Conversion1/1
  Gain2/1 -> Data Type Conversion6/1
  Gain4/1 -> Data Type Conversion7/1

== system UserBlocks/TTS Steering Control/Compute Steering Along Path/StaticMap/Map-Matching Primatives Dynamic Map P1/General Map-Matching Dynamic Map/Get Segment Info Dynamic Map ==
  segmentNumber : Inport
  Map : Inport  Port=2
  Bus Creator : BusCreator  Inputs=16
  Bus Selector : BusSelector  OutputSignals=segType,segLength,cumLength,Einit,Ninit,Uinit,psiInit,kStart,kEnd,grade,bank,maxE,maxV,fricBase,segModType
  Selector{,1..14} (15 alike) : Selector  IndexMode=Zero-based  IndexOptions=Index vector (port)  Indices=[1 3]
  segInfo : Outport
  wires:
  Selector14/1 -> Bus Creator/16  "segModType"
  Bus Selector/15 -> Selector14/1  "<segModType>"
  Selector8/1 -> Bus Creator/10  "kEnd"
  Selector7/1 -> Bus Creator/9  "kStart"
  Selector6/1 -> Bus Creator/8  "psiInit"
  Selector5/1 -> Bus Creator/7  "Uinit"
  Selector4/1 -> Bus Creator/6  "Ninit"
  Selector3/1 -> Bus Creator/5  "Einit"
  Selector2/1 -> Bus Creator/4  "cumLength"
  Selector1/1 -> Bus Creator/3  "segLength"
  Selector/1 -> Bus Creator/2  "segType"
  Selector9/1 -> Bus Creator/11  "grade"
  Selector10/1 -> Bus Creator/12  "bank"
  Selector11/1 -> Bus Creator/13  "maxE"
  Selector12/1 -> Bus Creator/14  "maxV"
  Selector13/1 -> Bus Creator/15  "frictionBase"
  segmentNumber/1 -> Bus Creator/1, Selector10/2, Selector14/2, Selector13/2, Selector12/2, Selector11/2, Selector9/2, Selector8/2, Selector7/2, Selector6/2, Selector5/2, Selector4/2, Selector3/2, Selector2/2, Selector1/2, Selector/2  "segNum"
  Bus Selector/14 -> Selector13/1  "<fricBase>"
  Bus Selector/13 -> Selector12/1  "<maxV>"
  Bus Selector/12 -> Selector11/1  "<maxE>"
  Bus Selector/11 -> Selector10/1  "<bank>"
  Bus Selector/10 -> Selector9/1  "<grade>"
  Bus Selector/9 -> Selector8/1  "<kEnd>"
  Bus Selector/8 -> Selector7/1  "<kStart>"
  Bus Selector/7 -> Selector6/1  "<psiInit>"
  Bus Selector/6 -> Selector5/1  "<Uinit>"
  Bus Selector/5 -> Selector4/1  "<Ninit>"
  Bus Selector/4 -> Selector3/1  "<Einit>"
  Bus Selector/3 -> Selector2/1  "<cumLength>"
  Bus Selector/2 -> Selector1/1  "<segLength>"
  Bus Selector/1 -> Selector/1  "<segType>"
  Map/1 -> Bus Selector/1
  Bus Creator/1 -> segInfo/1

== system UserBlocks/TTS Steering Control/Compute Steering Along Path/StaticMap/Map-Matching Primatives Dynamic Map P1/General Map-Matching Dynamic Map/mapMatchingPrimitives Dynamic Map ==
  posE : Inport
  posN : Inport  Port=2
  yawAngle : Inport  Port=3
  enable : Inport  Port=4
  Map : Inport  Port=5
  Bus Selector : BusSelector  OutputSignals=totalSegs,mapType,totalLength,segLength,cumLength,Einit,Ninit,psiInit,kStart,kEnd
  Constant : Constant  Value=mapMatchingParams
  Delay1 : TransportDelay  DelayTime=Ts
  Delay3 : TransportDelay  DelayTime=Ts  InitialOutput=-1
  Embedded MATLAB Function : MATLAB Function  TreatAsAtomicUnit=on
  Mux : Mux  Inputs=6
  SoE{,1..10} (11 alike) : Sum  Inputs=+
  zErr : Constant  Value=0
  seg : Outport
  e : Outport  Port=2
  deltaPsi : Outport  Port=3
  curvature : Outport  Port=4
  distanceToEnd : Outport  Port=5
  currentSegmentProgress : Outport  Port=6
  isFinalSegment : Outport  Port=7
  debugOut : Outport  Port=8
  wires:
  SoE5/1 -> Mux/5, Delay3/1
  SoE9/1 -> Mux/2
  SoE8/1 -> Mux/1
  SoE7/1 -> currentSegmentProgress/1
  SoE6/1 -> seg/1, Delay1/1
  SoE3/1 -> isFinalSegment/1
  Embedded MATLAB Function/6(s) -> SoE5/1  "s"
  Embedded MATLAB Function/1(e) -> SoE/1  "e"
  posE/1 -> Embedded MATLAB Function/1(posE)
  posN/1 -> Embedded MATLAB Function/2(posN)
  yawAngle/1 -> Embedded MATLAB Function/3(yawAngle)
  Constant/1 -> Embedded MATLAB Function/5(mapMatchingParams)
  Embedded MATLAB Function/7(seg) -> SoE6/1
  Embedded MATLAB Function/5(distanceToEnd) -> SoE4/1  "distanceToEnd"
  Embedded MATLAB Function/8(currentSegmentProgress) -> SoE7/1
  Embedded MATLAB Function/9(iterationCount) -> SoE8/1  "iterationCount"
  Embedded MATLAB Function/10(wasMax) -> SoE9/1  "wasMax"
  Embedded MATLAB Function/11(deltaS) -> SoE10/1  "resErr"
  zErr/1 -> Mux/6  "zErr"
  Mux/1 -> debugOut/1
  enable/1 -> Embedded MATLAB Function/4(enable), Mux/4  "enable"
  SoE4/1 -> distanceToEnd/1
  SoE10/1 -> Mux/3
  Embedded MATLAB Function/3(curvature) -> SoE2/1  "curvature"
  Embedded MATLAB Function/2(deltaPsi) -> SoE1/1  "deltaPsi"
  Embedded MATLAB Function/4(isFinalSegment) -> SoE3/1  "isFinalSegment"
  SoE2/1 -> curvature/1
  SoE1/1 -> deltaPsi/1
  SoE/1 -> e/1
  Delay1/1 -> Embedded MATLAB Function/17(prevSeg)
  Delay3/1 -> Embedded MATLAB Function/16(prevDist)
  Map/1 -> Bus Selector/1
  Bus Selector/1 -> Embedded MATLAB Function/6(totalSegs)  "<totalSegs>"
  Bus Selector/2 -> Embedded MATLAB Function/7(mapIsOpen)  "<mapType>"
  Bus Selector/3 -> Embedded MATLAB Function/8(totalMapLength)  "<totalLength>"
  Bus Selector/4 -> Embedded MATLAB Function/9(segLength)  "<segLength>"
  Bus Selector/5 -> Embedded MATLAB Function/10(cumulativeLength)  "<cumLength>"
  Bus Selector/6 -> Embedded MATLAB Function/11(EInit)  "<Einit>"
  Bus Selector/7 -> Embedded MATLAB Function/12(NInit)  "<Ninit>"
  Bus Selector/8 -> Embedded MATLAB Function/13(psiInit)  "<psiInit>"
  Bus Selector/9 -> Embedded MATLAB Function/14(kStart)  "<kStart>"
  Bus Selector/10 -> Embedded MATLAB Function/15(kEnd)  "<kEnd>"

== matlab function UserBlocks/TTS Steering Control/Compute Steering Along Path/StaticMap/MATLAB Function ==
  data: mapData input; segNum output; segType output; segLength output; cumLength output; Einit output; Ninit output; Uinit output; psiInit output; kStart output; kEnd output; grade output; bank output; maxE output; maxV output; fricBase output; fricUpdated output; segModType output; mapType output; totalLength output; totalSegs output
function [segNum,segType,segLength,cumLength,Einit,Ninit,Uinit,psiInit,kStart,kEnd,grade,bank,maxE,maxV,fricBase,fricUpdated,segModType,mapType, totalLength, totalSegs]= fcn(mapData)
%#codegen

segNum =        mapData(:,1);
segLength =     mapData(:,2); 
cumLength =     mapData(:,3); 
Einit =         mapData(:,4); 
Ninit =         mapData(:,5);
Uinit =         mapData(:,6); 
psiInit =       mapData(:,7); 
kStart =        mapData(:,8); 
kEnd =          mapData(:,9); 
grade =         mapData(:,10);
bank =          mapData(:,11); 
maxE =          mapData(:,12); 
maxV =          mapData(:,13);
fricBase =      mapData(:,14); 
fricUpdated =   mapData(:,15);  

mapType =       mapData(1,16);
totalLength =   mapData(1,17);
totalSegs =     mapData(1,18);


segType =       zeros(length(segNum),1)-1; % initialize
segModType =    zeros(length(segNum),1)-1; % initialize

%coder.varsize('segModType',[length(segNum) 1])
%segModType = 1;
for i=1:totalSegs
    
    % seg modification type - 0 states that its the original
    segModType(i) = 0;
   
    % seg type - what kind of segment each is
    if kEnd(i)==kStart(i) && kEnd(i)==0
        segType(i) = 0; % straight
    elseif abs(kEnd(i))>abs(kStart(i))
        segType(i) = 1; % entry clothoid
    elseif abs(kEnd(i))<abs(kStart(i))
        segType(i) = 3; % exit clothoid
    elseif kEnd(i)==kStart(i) && kEnd(i)~=0 && kEnd(i)~=-1
        segType(i) = 2; % const radius        
    else
        segType(i) = -1; % we have a problem        
    end
    
end
